simulink model "ECS_Fight_Control_System - Final"  (R2025a)
settings: Solver=ode15s  StartTime=0.0  StopTime=5000  MaxStep=0.1  RelTol=1e-2
libraries: fl_lib x34, nesl_utility x18, SimscapeFluids_lib x8, batt_lib x3, simulink x3, slpidlib x3, simulink_extras x1
(part 1 of 2)
settings Model: SimulationMode=accelerator  Creator=Piyusha  LastModifiedBy=Piyusha

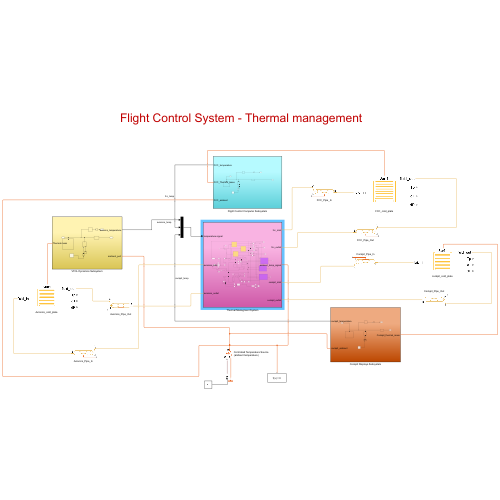
[thumbnail: Simulink's stored preview of the top-level diagram]
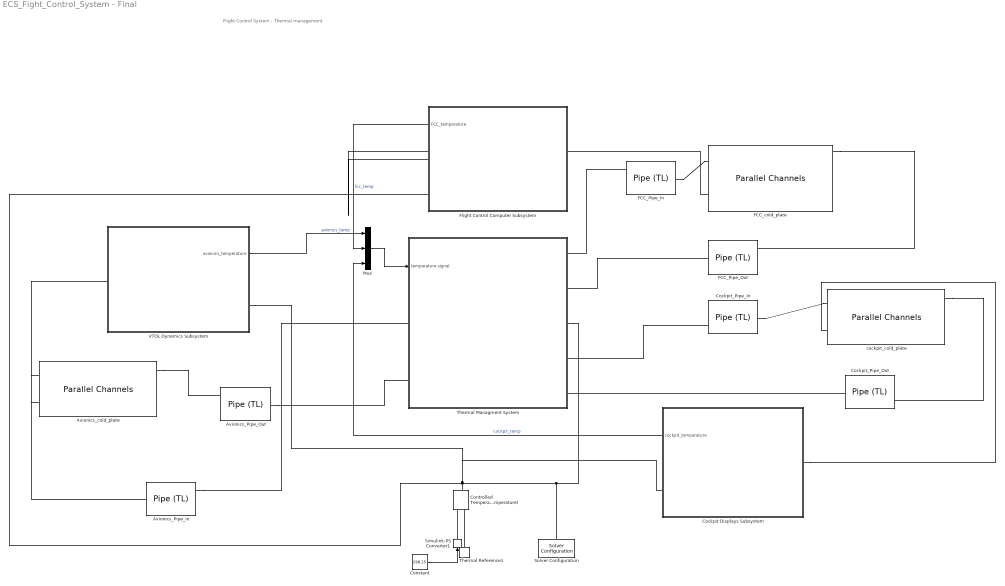
== system ECS_Fight_Control_System - Final ==
  note: Flight Control System - Thermal management
  Avionics_Pipe_In : fl_lib/Thermal Liquid/Elements/Pipe (TL)  length=0.5 m  area=0.006 m^2  Dh=2.827e-5 m  length_add=1 m  roughness=15e-6 m  Re_lam=2000  Re_tur=4000  shape_factor=64  Nu_lam=3.66  dynamic_compressibility=true  inertia=false  p0=0.101325 MPa  T0=298.15 K  mdot0=0 kg/s  p_nominal=0.101325 MPa  T_nominal=293.15 K
  Avionics_Pipe_Out : fl_lib/Thermal Liquid/Elements/Pipe (TL)  length=0.5 m  area=0.006 m^2  Dh=2.827e-5 m  length_add=1 m  roughness=15e-6 m  Re_lam=2000  Re_tur=4000  shape_factor=64  Nu_lam=3.66  dynamic_compressibility=true  inertia=false  p0=0.101325 MPa  T0=298.15 K  mdot0=0 kg/s  p_nominal=0.101325 MPa  T_nominal=293.15 K
  Avionics_cold_plate : batt_lib/Thermal/Parallel Channels  plateConnectivity=simscape.battery.enum.thermal.coolingPlateConnectivity.singleSided  numBattThermalNodes1=1  dimensionThermalNodes1=ones(1, 2)  locationThermalNodes1=ones(1, 2)  numBattThermalNodes2=1  dimensionThermalNodes2=ones(1, 2)  locationThermalNodes2=ones(1, 2)  plateDimX=2  plateDimY=5  plateTh=3e-3 m  plateThCond=200 W/(K*m)  plateDen=2700 kg/m^3  plateCp=900 J/(K*kg)  plateTemp_ini=298.15 K  Re_lam=2000  Re_tur=4000  Nu_lam=3.66  length_add=1e-3 m  shape_factor=64  nChannels=10  selectChannelOrientation=simscape.battery.enum.thermal.coolingChannelsDirection.alongX  channelDia=0.005 m  distributorDia=0.005 m  roughnessPipe=1.5e-05 m
      settings: InternalSimscapePortConfiguration="{\"Bottom\":[],\"Left\":[{\"id\":\"fluid_in\",\"label\":\"fluid_in\",\"type\":\"foundation.thermal_liquid.thermal_liquid\"}],\"Right\":[{\"id\":\"fluid_out\",\"label\":\"fluid_out\",\"type\":\"foundation.thermal_liquid.thermal_liquid\"},{\"id\":\"plotPlateT\",\"label\":\"Tp\",\"type\":\"output\"},{\"id\":\"tempSensor\",\"label\":\"dT\",\"type\":\"output\"},{\"id\":\"presSensor\",\"label\":\"dP\",\"type\":\"output\"}],\"Top\":[{\"id\":\"Side1\",\"label\":\"Surf1\",\"type\":\"foundation.thermal.thermal\"}]}"
  Cockpit Displays Subsystem : Subsystem
  Cockpit_Pipe_In : fl_lib/Thermal Liquid/Elements/Pipe (TL)  length=0.5 m  area=0.006 m^2  Dh=2.827e-5 m  length_add=1 m  roughness=15e-6 m  Re_lam=2000  Re_tur=4000  shape_factor=64  Nu_lam=3.66  dynamic_compressibility=true  inertia=false  p0=0.101325 MPa  T0=298.15 K  mdot0=0 kg/s  p_nominal=0.101325 MPa  T_nominal=293.15 K
  Cockpit_Pipe_Out : fl_lib/Thermal Liquid/Elements/Pipe (TL)  length=0.5 m  area=0.006 m^2  Dh=2.827e-5 m  length_add=1 m  roughness=15e-6 m  Re_lam=2000  Re_tur=4000  shape_factor=64  Nu_lam=3.66  dynamic_compressibility=true  inertia=false  p0=0.101325 MPa  T0=298.15 K  mdot0=0 kg/s  p_nominal=0.101325 MPa  T_nominal=293.15 K
  Constant : Constant  Value=298.15
  Controlled Temperature Source (ambient temperature) : fl_lib/Thermal/Thermal Sources/Controlled Temperature Source
  FCC_Pipe_In : fl_lib/Thermal Liquid/Elements/Pipe (TL)  length=0.5 m  area=0.006 m^2  Dh=2.827e-5 m  length_add=1 m  roughness=15e-6 m  Re_lam=2000  Re_tur=4000  shape_factor=64  Nu_lam=3.66  dynamic_compressibility=true  inertia=false  p0=0.101325 MPa  T0=298.15 K  mdot0=0 kg/s  p_nominal=0.101325 MPa  T_nominal=293.15 K
  FCC_Pipe_Out : fl_lib/Thermal Liquid/Elements/Pipe (TL)  length=0.5 m  area=0.006 m^2  Dh=2.827e-5 m  length_add=1 m  roughness=15e-6 m  Re_lam=2000  Re_tur=4000  shape_factor=64  Nu_lam=3.66  dynamic_compressibility=true  inertia=false  p0=0.101325 MPa  T0=298.15 K  mdot0=0 kg/s  p_nominal=0.101325 MPa  T_nominal=293.15 K
  FCC_cold_plate : batt_lib/Thermal/Parallel Channels  plateConnectivity=simscape.battery.enum.thermal.coolingPlateConnectivity.singleSided  numBattThermalNodes1=1  dimensionThermalNodes1=ones(1, 2)  locationThermalNodes1=ones(1, 2)  numBattThermalNodes2=1  dimensionThermalNodes2=ones(1, 2)  locationThermalNodes2=ones(1, 2)  plateDimX=2  plateDimY=5  plateTh=3e-3 m  plateThCond=200 W/(K*m)  plateDen=2700 kg/m^3  plateCp=900 J/(K*kg)  plateTemp_ini=298.15 K  Re_lam=2000  Re_tur=4000  Nu_lam=3.66  length_add=1e-3 m  shape_factor=64  nChannels=16  selectChannelOrientation=simscape.battery.enum.thermal.coolingChannelsDirection.alongX  channelDia=0.005 m  distributorDia=0.005 m  roughnessPipe=1.5e-05 m
      settings: InternalSimscapePortConfiguration="{\"Bottom\":[],\"Left\":[{\"id\":\"fluid_in\",\"label\":\"fluid_in\",\"type\":\"foundation.thermal_liquid.thermal_liquid\"}],\"Right\":[{\"id\":\"fluid_out\",\"label\":\"fluid_out\",\"type\":\"foundation.thermal_liquid.thermal_liquid\"},{\"id\":\"plotPlateT\",\"label\":\"Tp\",\"type\":\"output\"},{\"id\":\"tempSensor\",\"label\":\"dT\",\"type\":\"output\"},{\"id\":\"presSensor\",\"label\":\"dP\",\"type\":\"output\"}],\"Top\":[{\"id\":\"Side1\",\"label\":\"Surf1\",\"type\":\"foundation.thermal.thermal\"}]}"
  Flight Control Computer Subsystem : Subsystem
  Mux : Mux  Inputs=3
  Simulink-PS Converter1 : nesl_utility/Simulink-PS Converter  PhysicalDomain=network_engine_domain  SubClassName=ps_input  LeftPortType=input  RightPortType=output  PseudoPeriodic=off  Frequencies=[]  NoiseDistribution=none  NoiseParameters=[]  Unit=K  AffineConversion=off  FilteringAndDerivatives=provide  SimscapeFilterOrder=1  InputFilterTimeConstant=0.001  UdotUserProvided=0
  Solver Configuration : nesl_utility/Solver Configuration  PhysicalDomain=network_engine_domain  SubClassName=solver  LeftPortType=input  RightPortType=generic  Tones=[]  Harmonics=[]  SimulateNoise=off  Profile=off  UseLocalSampling=off  EnableSwitchedLinearOptims=on  FrequencyDomain=off  UseCCode=off  RelTol=0.001  AbsTol=0.001  MinStep=1e-09  ToWorkspace=off  RevertToSquareIcSolve=off  NumHomotopyIterations=100  PhasorMode=off  PhasorModeNumHarmonics=1  ConsistencySolver=NEWTON_XTOL_AFTER_FTOL  IndexReductionMethod=DerivativeReplacement  DoDC=off  ResidualTolerance=1e-09  ConsistencyTolSource=GLOBAL  ConsistencyAbsTol=0.001  ConsistencyRelTol=0.001  ConsistencyTolFactor=0.001  UseLocalSolver=off  LocalSolverChoice=NE_BACKWARD_EULER_ADVANCER  ResolveIndetEquations=on  FunctionEvalNumThread=1  LocalSolverSampleTime=0.001  DoFixedCost=off  MaxNonlinIter=3  MaxModeIter=2  ComputeImpulses=off  ImpulseIterations=2  LinearAlgebra=auto  LinearAlgebraNumThread=0  EquationFormulation=NE_TIME_EF  DelaysMemoryBudget=1024  AutomaticFiltering=on  FilteringTimeConstant=0.001  PartitionStorageMethod=AS_NEEDED  PartitionMemoryBudget=1024  PartitionMethod=ROBUST  MultibodyUseLocalSolver=off  MultibodyLocalSolverChoice=ODE1  MultibodyLocalSolverSampleTime=0.001
  Thermal Managment System : Subsystem
  Thermal Reference1 : fl_lib/Thermal/Thermal Elements/Thermal Reference
  VTOL Dynamics Subsystem : Subsystem
  cockpit_cold_plate : batt_lib/Thermal/Parallel Channels  plateConnectivity=simscape.battery.enum.thermal.coolingPlateConnectivity.singleSided  numBattThermalNodes1=1  dimensionThermalNodes1=ones(1, 2)  locationThermalNodes1=ones(1, 2)  numBattThermalNodes2=1  dimensionThermalNodes2=ones(1, 2)  locationThermalNodes2=ones(1, 2)  plateDimX=2  plateDimY=5  plateTh=3e-3 m  plateThCond=200 W/(K*m)  plateDen=2700 kg/m^3  plateCp=900 J/(K*kg)  plateTemp_ini=298.15 K  Re_lam=2000  Re_tur=4000  Nu_lam=3.66  length_add=1e-3 m  shape_factor=64  nChannels=24  selectChannelOrientation=simscape.battery.enum.thermal.coolingChannelsDirection.alongX  channelDia=0.005 m  distributorDia=0.005 m  roughnessPipe=1.5e-05 m
      settings: InternalSimscapePortConfiguration="{\"Bottom\":[],\"Left\":[{\"id\":\"fluid_in\",\"label\":\"fluid_in\",\"type\":\"foundation.thermal_liquid.thermal_liquid\"}],\"Right\":[{\"id\":\"fluid_out\",\"label\":\"fluid_out\",\"type\":\"foundation.thermal_liquid.thermal_liquid\"},{\"id\":\"plotPlateT\",\"label\":\"Tp\",\"type\":\"output\"},{\"id\":\"tempSensor\",\"label\":\"dT\",\"type\":\"output\"},{\"id\":\"presSensor\",\"label\":\"dP\",\"type\":\"output\"}],\"Top\":[{\"id\":\"Side1\",\"label\":\"Surf1\",\"type\":\"foundation.thermal.thermal\"}]}"
  wires:
  Flight Control Computer Subsystem/1(FCC_temperature) -> Mux/2  "fcc_temp"
  Cockpit Displays Subsystem/1(cockpit_temperature) -> Mux/3  "cockpit_temp"
  VTOL Dynamics Subsystem/1(avionics_temperature) -> Mux/1  "avionics_temp"
  Mux/1 -> Thermal Managment System/1(temperature signal)
  Constant/1 -> Simulink-PS Converter1/1
  connections:
  Thermal Reference1/LConn1 -- Controlled Temperature Source (ambient temperature)/RConn2
  Simulink-PS Converter1/RConn1 -- Controlled Temperature Source (ambient temperature)/RConn1
  Thermal Managment System/RConn3 -- VTOL Dynamics Subsystem/RConn1 -- Cockpit Displays Subsystem/RConn1 -- Controlled Temperature Source (ambient temperature)/LConn1 -- Flight Control Computer Subsystem/RConn2 -- Solver Configuration/RConn1
  Avionics_cold_plate/LConn2 -- VTOL Dynamics Subsystem/LConn1
  Avionics_Pipe_In/RConn1 -- Avionics_cold_plate/LConn1
  Avionics_cold_plate/RConn1 -- Avionics_Pipe_Out/LConn1
  Avionics_Pipe_In/LConn1 -- Thermal Managment System/LConn1
  Avionics_Pipe_Out/RConn1 -- Thermal Managment System/LConn2
  FCC_Pipe_In/RConn1 -- FCC_cold_plate/LConn1
  FCC_cold_plate/RConn1 -- FCC_Pipe_Out/LConn1
  FCC_Pipe_In/LConn1 -- Thermal Managment System/RConn1
  FCC_Pipe_Out/RConn1 -- Thermal Managment System/RConn2
  Cockpit_Pipe_In/RConn1 -- cockpit_cold_plate/LConn1
  cockpit_cold_plate/RConn1 -- Cockpit_Pipe_Out/LConn1
  Cockpit_Pipe_In/LConn1 -- Thermal Managment System/RConn4
  Cockpit_Pipe_Out/RConn1 -- Thermal Managment System/RConn5
  Cockpit Displays Subsystem/LConn1 -- cockpit_cold_plate/LConn2
  FCC_cold_plate/LConn2 -- Flight Control Computer Subsystem/RConn1

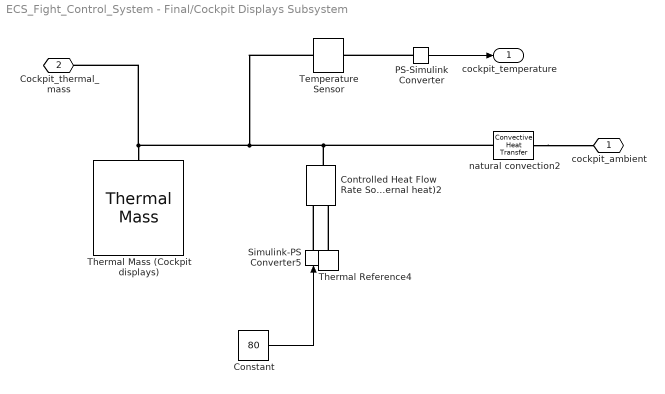
== system ECS_Fight_Control_System - Final/Cockpit Displays Subsystem ==
  Constant : Constant  Value=80
  Controlled Heat Flow Rate Source (Internal heat)2 : fl_lib/Thermal/Thermal Sources/Controlled Heat Flow Rate Source
  PS-Simulink Converter : nesl_utility/PS-Simulink Converter  PhysicalDomain=network_engine_domain  SubClassName=ps_output  LeftPortType=input  RightPortType=output  PseudoPeriodic=off  Frequencies=[]  VectorFormat=inherit  Unit=inherit  AffineConversion=off
  Simulink-PS Converter5 : nesl_utility/Simulink-PS Converter  PhysicalDomain=network_engine_domain  SubClassName=ps_input  LeftPortType=input  RightPortType=output  PseudoPeriodic=off  Frequencies=[]  NoiseDistribution=none  NoiseParameters=[]  Unit=W  AffineConversion=off  FilteringAndDerivatives=provide  SimscapeFilterOrder=1  InputFilterTimeConstant=0.001  UdotUserProvided=0
  Temperature Sensor : fl_lib/Thermal/Thermal Sensors/Temperature Sensor  temperature_measure=foundation.enum.MeasurementReference.absolute
      settings: InternalSimscapePortConfiguration="{\"Bottom\":[],\"Left\":[{\"id\":\"A\",\"label\":\"A\",\"type\":\"foundation.thermal.thermal\"}],\"Right\":[{\"id\":\"T\",\"label\":\"T\",\"type\":\"output\"}],\"Top\":[]}"
  Thermal Mass (Cockpit displays) : fl_lib/Thermal/Thermal Elements/Thermal Mass  mass_type=foundation.enum.constant_variable.constant  mass=13 kg  sp_heat=900 J/(K*kg)  mass_min=1e-6 kg  num_ports=foundation.enum.numPorts2.one  m_specify=off  m_priority=High  m=1 kg  m_nominal_specify=off  m_nominal_value=1  m_nominal_unit=kg  T_specify=on  T_priority=None  T=312 K  T_nominal_specify=off  T_nominal_value=350  T_nominal_unit=K  Q_specify=off  Q_priority=None  Q=0 W  Q_nominal_specify=off  Q_nominal_value=1  Q_nominal_unit=W
  Thermal Reference4 : fl_lib/Thermal/Thermal Elements/Thermal Reference
  natural convection2 : fl_lib/Thermal/Thermal Elements/Convective Heat Transfer  thermal_type=foundation.enum.constant_variable.constant  area=0.3 m^2  heat_tr_coeff=10 W/(K*m^2)  min_heat_tr_coeff=1e-3 W/(K*m^2)  T_specify=off  T_priority=None  T=0 K  T_nominal_specify=off  T_nominal_value=1  T_nominal_unit=K  Q_specify=off  Q_priority=None  Q=0 W  Q_nominal_specify=off  Q_nominal_value=1  Q_nominal_unit=W
  cockpit_ambient : PMIOPort  Side=Right
  Cockpit_thermal_mass : PMIOPort  Port=2  Side=Left
  cockpit_temperature : Outport
  wires:
  PS-Simulink Converter/1 -> cockpit_temperature/1
  Constant/1 -> Simulink-PS Converter5/1
  connections:
  natural convection2/RConn1 -- cockpit_ambient/RConn1
  Controlled Heat Flow Rate Source (Internal heat)2/LConn1 -- natural convection2/LConn1 -- Temperature Sensor/LConn1 -- Cockpit_thermal_mass/RConn1 -- Thermal Mass (Cockpit displays)/LConn1
  Simulink-PS Converter5/RConn1 -- Controlled Heat Flow Rate Source (Internal heat)2/RConn1
  Thermal Reference4/LConn1 -- Controlled Heat Flow Rate Source (Internal heat)2/RConn2
  PS-Simulink Converter/LConn1 -- Temperature Sensor/RConn1

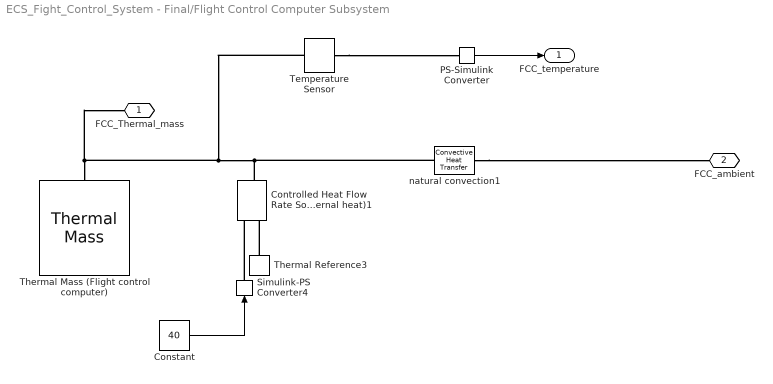
== system ECS_Fight_Control_System - Final/Flight Control Computer Subsystem ==
  Constant : Constant  Value=40
  Controlled Heat Flow Rate Source (Internal heat)1 : fl_lib/Thermal/Thermal Sources/Controlled Heat Flow Rate Source
  PS-Simulink Converter : nesl_utility/PS-Simulink Converter  PhysicalDomain=network_engine_domain  SubClassName=ps_output  LeftPortType=input  RightPortType=output  PseudoPeriodic=off  Frequencies=[]  VectorFormat=inherit  Unit=inherit  AffineConversion=off
  Simulink-PS Converter4 : nesl_utility/Simulink-PS Converter  PhysicalDomain=network_engine_domain  SubClassName=ps_input  LeftPortType=input  RightPortType=output  PseudoPeriodic=off  Frequencies=[]  NoiseDistribution=none  NoiseParameters=[]  Unit=W  AffineConversion=off  FilteringAndDerivatives=provide  SimscapeFilterOrder=1  InputFilterTimeConstant=0.001  UdotUserProvided=0
  Temperature Sensor : fl_lib/Thermal/Thermal Sensors/Temperature Sensor  temperature_measure=foundation.enum.MeasurementReference.absolute
      settings: InternalSimscapePortConfiguration="{\"Bottom\":[],\"Left\":[{\"id\":\"A\",\"label\":\"A\",\"type\":\"foundation.thermal.thermal\"}],\"Right\":[{\"id\":\"T\",\"label\":\"T\",\"type\":\"output\"}],\"Top\":[]}"
  Thermal Mass (Flight control computer) : fl_lib/Thermal/Thermal Elements/Thermal Mass  mass_type=foundation.enum.constant_variable.constant  mass=4.5 kg  sp_heat=900 J/(K*kg)  mass_min=1e-6 kg  num_ports=foundation.enum.numPorts2.one  m_specify=off  m_priority=High  m=1 kg  m_nominal_specify=off  m_nominal_value=1  m_nominal_unit=kg  T_specify=on  T_priority=None  T=310 K  T_nominal_specify=off  T_nominal_value=350  T_nominal_unit=K  Q_specify=off  Q_priority=None  Q=0 W  Q_nominal_specify=off  Q_nominal_value=1  Q_nominal_unit=W
  Thermal Reference3 : fl_lib/Thermal/Thermal Elements/Thermal Reference
  natural convection1 : fl_lib/Thermal/Thermal Elements/Convective Heat Transfer  thermal_type=foundation.enum.constant_variable.constant  area=0.22 m^2  heat_tr_coeff=10 W/(K*m^2)  min_heat_tr_coeff=1e-3 W/(K*m^2)  T_specify=off  T_priority=None  T=0 K  T_nominal_specify=off  T_nominal_value=1  T_nominal_unit=K  Q_specify=off  Q_priority=None  Q=0 W  Q_nominal_specify=off  Q_nominal_value=1  Q_nominal_unit=W
  FCC_Thermal_mass : PMIOPort  Side=Right
  FCC_ambient : PMIOPort  Port=2  Side=Right
  FCC_temperature : Outport
  wires:
  PS-Simulink Converter/1 -> FCC_temperature/1
  Constant/1 -> Simulink-PS Converter4/1
  connections:
  Thermal Reference3/LConn1 -- Controlled Heat Flow Rate Source (Internal heat)1/RConn2
  Simulink-PS Converter4/RConn1 -- Controlled Heat Flow Rate Source (Internal heat)1/RConn1
  natural convection1/LConn1 -- Temperature Sensor/LConn1 -- FCC_Thermal_mass/RConn1 -- Thermal Mass (Flight control computer)/LConn1 -- Controlled Heat Flow Rate Source (Internal heat)1/LConn1
  natural convection1/RConn1 -- FCC_ambient/RConn1
  Temperature Sensor/RConn1 -- PS-Simulink Converter/LConn1

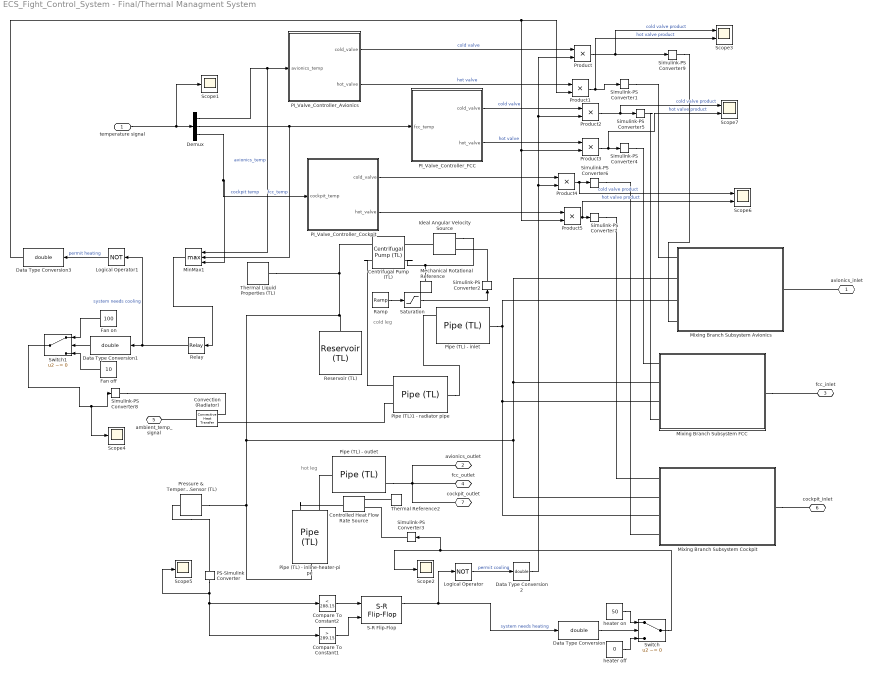
== system ECS_Fight_Control_System - Final/Thermal Managment System ==
  note: cold leg
  note: hot leg
  temperature signal : Inport
  Centrifugal Pump (TL) : SimscapeFluids_lib/Thermal Liquid/Pumps & Motors/Centrifugal Pump (TL)  pump_parameterization=fluids.thermal_liquid.pumps_motors.enum.CentrifugalPumpParameterization.Nominal  capacity_ref_nominal=5 lpm  head_ref_nominal=4 m  power_ref_nominal=0.02 kW  head_ref_max=8 m  capacity_ref_max=8 lpm  omega_ref_analytic=3000 rpm  flow_rate_1D_TLU=[16.67, 30, 40, 53.33, 66.67, 83.33] lpm  head_1D_TLU=[50, 47.5, 45, 40, 35, 25] m  power_1D_TLU=[.6, .75, .85, .93, .98, .99] kW  omega_ref_1D=3500 rpm  rho_ref_1D=998.21 kg/m^3  omega_threshold_factor=1e-2  flow_rate_2D_TLU=[16.67, 23.33, 30, 40, 53.33, 60] lpm  omega_2D_TLU=[2450, 2800, 3150, 3500] rpm  head_2D_TLU=[25, 32.7, 42.5, 50; 24, 31.7, 41, 49; 22.7, 30.5, 39, 47.5; 20, 28, 36, 45; 15.7, 24, 32, 40; 12.5, 21, 29.5, 37.5] m  power_2D_TLU=[.28, .38, .5, .6; .31, .41, .55, .68; .33, .44, .6, .75; .36, .48, .65, .83; .38, .53, .72, .93; .39, .55, .75, .97] kW  rho_ref_2D=998.21 kg/m^3  diameter_ratio=1  mech_orientation=fluids.thermal_liquid.pumps_motors.enum.CentrifugalPumpMechOrientation.Positive  area=7.854e-5 m^2  operation_check=simscape.enum.assert.action.none
      settings: InternalSimscapePortConfiguration="{\"Bottom\":[],\"Left\":[{\"id\":\"A\",\"label\":\"A\",\"type\":\"foundation.thermal_liquid.thermal_liquid\"},{\"id\":\"B\",\"label\":\"B\",\"type\":\"foundation.thermal_liquid.thermal_liquid\"}],\"Right\":[{\"id\":\"R\",\"label\":\"R\",\"type\":\"foundation.mechanical.rotational.rotational\"},{\"id\":\"C\",\"label\":\"C\",\"type\":\"foundation.mechanical.rotational.rotational\"}],\"Top\":[]}"
  Compare To Constant1 : simulink/Logic and Bit Operations/Compare To Constant  relop=>  const=289.15  OutDataTypeStr=boolean
  Compare To Constant2 : simulink/Logic and Bit Operations/Compare To Constant  relop=<  const=288.15  OutDataTypeStr=boolean
  Controlled Heat Flow Rate Source : fl_lib/Thermal/Thermal Sources/Controlled Heat Flow Rate Source
  Convection (Radiator) : fl_lib/Thermal/Thermal Elements/Convective Heat Transfer  thermal_type=foundation.enum.constant_variable.variable  area=0.5 m^2  heat_tr_coeff=100 W/(K*m^2)  min_heat_tr_coeff=1e-3 W/(K*m^2)  T_specify=off  T_priority=None  T=0 K  T_nominal_specify=off  T_nominal_value=1  T_nominal_unit=K  Q_specify=off  Q_priority=None  Q=0 W  Q_nominal_specify=off  Q_nominal_value=1  Q_nominal_unit=W
      settings: InternalSimscapePortConfiguration="{\"Bottom\":[],\"Left\":[{\"id\":\"A\",\"label\":\"A\",\"type\":\"foundation.thermal.thermal\"},{\"id\":\"var_heat_tr_coeff\",\"label\":\"K\",\"type\":\"input\"}],\"Right\":[{\"id\":\"B\",\"label\":\"B\",\"type\":\"foundation.thermal.thermal\"}],\"Top\":[]}"
  Data Type Conversion{,1..3} (4 alike) : DataTypeConversion  OutDataTypeStr=double  SaturateOnIntegerOverflow=off  RndMeth=Floor
  Demux : Demux  Outputs=3
  Fan off : Constant  Value=10
  Fan on : Constant  Value=100
  Ideal Angular Velocity Source : fl_lib/Mechanical/Mechanical Sources/Ideal Angular Velocity Source
  Logical Operator : Logic  Operator=NOT  AllPortsSameDT=off  OutDataTypeStr=boolean
  Logical Operator1 : Logic  Operator=NOT  AllPortsSameDT=off  OutDataTypeStr=boolean
  Mechanical Rotational Reference : fl_lib/Mechanical/Rotational Elements/Mechanical Rotational Reference
  MinMax1 : MinMax  Function=max  Inputs=3
  Mixing Branch Subsystem Avionics : Subsystem
  Mixing Branch Subsystem Cockpit : Subsystem
  Mixing Branch Subsystem FCC : Subsystem
  PI_Valve_Controller_Avionics : Subsystem
  PI_Valve_Controller_Cockpit : Subsystem
  PI_Valve_Controller_FCC : Subsystem
  PS-Simulink Converter : nesl_utility/PS-Simulink Converter  PhysicalDomain=network_engine_domain  SubClassName=ps_output  LeftPortType=input  RightPortType=output  PseudoPeriodic=off  Frequencies=[]  VectorFormat=inherit  Unit=inherit  AffineConversion=off
  Pipe (TL) - inlet : fl_lib/Thermal Liquid/Elements/Pipe (TL)  length=1.5 m  area=7.854e-5 m^2  Dh=0.01 m  length_add=1 m  roughness=15e-6 m  Re_lam=2000  Re_tur=4000  shape_factor=64  Nu_lam=3.66  dynamic_compressibility=true  inertia=false  p0=0.101325 MPa  T0=298.15 K  mdot0=0 kg/s  p_nominal=0.101325 MPa  T_nominal=293.15 K
  Pipe (TL) - inline-heater-pipe : fl_lib/Thermal Liquid/Elements/Pipe (TL)  length=0.1 m  area=7.854e-5 m^2  Dh=0.01 m  length_add=1 m  roughness=15e-6 m  Re_lam=2000  Re_tur=4000  shape_factor=64  Nu_lam=3.66  dynamic_compressibility=true  inertia=false  p0=0.101325 MPa  T0=298.15 K  mdot0=0 kg/s  p_nominal=0.101325 MPa  T_nominal=293.15 K
  Pipe (TL) - outlet : fl_lib/Thermal Liquid/Elements/Pipe (TL)  length=1.5 m  area=7.854e-5 m^2  Dh=0.01 m  length_add=1 m  roughness=15e-6 m  Re_lam=2000  Re_tur=4000  shape_factor=64  Nu_lam=3.66  dynamic_compressibility=true  inertia=false  p0=0.101325 MPa  T0=298.15 K  mdot0=0 kg/s  p_nominal=0.101325 MPa  T_nominal=293.15 K
  Pipe (TL)1 - radiator pipe : fl_lib/Thermal Liquid/Elements/Pipe (TL)  length=0.75 m  area=7.854e-5 m^2  Dh=0.01 m  length_add=1 m  roughness=15e-6 m  Re_lam=2000  Re_tur=4000  shape_factor=64  Nu_lam=3.66  dynamic_compressibility=true  inertia=false  p0=0.101325 MPa  T0=298.15 K  mdot0=0 kg/s  p_nominal=0.101325 MPa  T_nominal=293.15 K
  Pressure & Temperature Sensor (TL) : fl_lib/Thermal Liquid/Sensors/Pressure & Temperature Sensor (TL)  reference=foundation.enum.MeasurementReference.absolute  pressure=false  pressure_spec=foundation.enum.PressureMeasementSpec.Absolute  temperature=true
      settings: InternalSimscapePortConfiguration="{\"Bottom\":[{\"id\":\"T\",\"label\":\"T\",\"type\":\"output\"}],\"Left\":[{\"id\":\"A\",\"label\":\"A\",\"type\":\"foundation.thermal_liquid.thermal_liquid\"}],\"Right\":[],\"Top\":[]}"
  Product{,1..5} (6 alike) : Product
  Ramp : simulink/Sources/Ramp  slope=1000  start=1  InitialOutput=0
  Relay : Relay  OnSwitchValue=308.15  OffSwitchValue=307.15
  "Reservoir (TL) " : fl_lib/Thermal Liquid/Elements/Reservoir (TL)  pressure_spec=foundation.enum.pressure_spec.atmospheric  reservoir_pressure=0.101325 MPa  reservoir_temperature=298.15 K  area=7.854e-5 m^2
  S-R Flip-Flop : simulink_extras/Flip Flops/S-R Flip-Flop  initial_condition=0
  Saturation : Saturate  UpperLimit=3000  LowerLimit=0
  Scope{1..2,4..5} (4 alike) : Scope
      Scope1 settings: ActiveDisplayYMinimum=294.34876570244938  ActiveDisplayYMaximum=309.81465883467445
      Scope2 settings: ActiveDisplayYMinimum=-18.574706388101248  ActiveDisplayYMaximum=67.656527037864834  DataLoggingVariableName=ScopeData2
      Scope4 settings: ActiveDisplayYMinimum=-17.443836096573261  ActiveDisplayYMaximum=62.456397666600694  DataLoggingVariableName=ScopeData4
      Scope5 settings: ActiveDisplayYMinimum=292.31370524419793  ActiveDisplayYMaximum=296.28099923951214  DataLoggingVariableName=ScopeData5
  Scope3 : Scope  NumInputPorts=2
      settings: ActiveDisplayYMinimum=-0.24217564391764534  ActiveDisplayYMaximum=0.68337651791294018  DataLoggingVariableName=ScopeData3
  Scope6 : Scope  NumInputPorts=2
      settings: ActiveDisplayYMinimum=-0.26550876950504732  ActiveDisplayYMaximum=1.3314895720023909  DataLoggingVariableName=ScopeData6
  Scope7 : Scope  NumInputPorts=2
      settings: ActiveDisplayYMinimum=-0.25040000463615819  ActiveDisplayYMaximum=1.2618169694914934
  Simulink-PS Converter{1,4..7,9} (6 alike) : nesl_utility/Simulink-PS Converter  PhysicalDomain=network_engine_domain  SubClassName=ps_input  LeftPortType=input  RightPortType=output  PseudoPeriodic=off  Frequencies=[]  NoiseDistribution=none  NoiseParameters=[]  Unit=1  AffineConversion=off  FilteringAndDerivatives=provide  SimscapeFilterOrder=1  InputFilterTimeConstant=0.001  UdotUserProvided=0
  Simulink-PS Converter2 : nesl_utility/Simulink-PS Converter  PhysicalDomain=network_engine_domain  SubClassName=ps_input  LeftPortType=input  RightPortType=output  PseudoPeriodic=off  Frequencies=[]  NoiseDistribution=none  NoiseParameters=[]  Unit=rpm  AffineConversion=off  FilteringAndDerivatives=provide  SimscapeFilterOrder=1  InputFilterTimeConstant=0.001  UdotUserProvided=0
  Simulink-PS Converter3 : nesl_utility/Simulink-PS Converter  PhysicalDomain=network_engine_domain  SubClassName=ps_input  LeftPortType=input  RightPortType=output  PseudoPeriodic=off  Frequencies=[]  NoiseDistribution=none  NoiseParameters=[]  Unit=W  AffineConversion=off  FilteringAndDerivatives=provide  SimscapeFilterOrder=1  InputFilterTimeConstant=0.001  UdotUserProvided=0
  Simulink-PS Converter8 : nesl_utility/Simulink-PS Converter  PhysicalDomain=network_engine_domain  SubClassName=ps_input  LeftPortType=input  RightPortType=output  PseudoPeriodic=off  Frequencies=[]  NoiseDistribution=none  NoiseParameters=[]  Unit=W/(m^2*K)  AffineConversion=off  FilteringAndDerivatives=provide  SimscapeFilterOrder=1  InputFilterTimeConstant=0.001  UdotUserProvided=0
  Switch : Switch  Criteria=u2 ~= 0  SaturateOnIntegerOverflow=off  InputSameDT=off
  Switch1 : Switch  Criteria=u2 ~= 0  SaturateOnIntegerOverflow=off  InputSameDT=off
  "Thermal Liquid Properties (TL) " : SimscapeFluids_lib/Thermal Liquid/Utilities/Thermal Liquid Properties (TL)  fluid_list=fluids.thermal_liquid.utilities.enum.thermal_liquid_fluid_list.ethylene_glycol  concentration_param_EG=fluids.thermal_liquid.utilities.enum.thermal_liquid_concentration.volume_fraction  concentration_param_PG=fluids.thermal_liquid.utilities.enum.thermal_liquid_concentration.volume_fraction  c_mass_SW=3.5e-3  c_mass_EG=0.1  c_mass_PG=0.1  c_mass_GL=0.1  c_vol_EG=0.6  c_vol_PG=0.1  beta_const_EG=2.1791 GPa  beta_const_PG=2.1791 GPa  beta_const_GL=2.1791 GPa  p_min_EG=0.01 MPa  p_min_PG=0.01 MPa  p_min_GL=0.01 MPa  p_max_EG=50 MPa  p_max_PG=50 MPa  p_max_GL=50 MPa  p_atm=0.101325 MPa  properties_range_check=simscape.enum.assert.action.error
  Thermal Reference2 : fl_lib/Thermal/Thermal Elements/Thermal Reference
  heater off : Constant  Value=0
  heater on : Constant  Value=50
  avionics_inlet : PMIOPort  Side=Left
  avionics_outlet : PMIOPort  Port=2  Side=Left
  fcc_inlet : PMIOPort  Port=3  Side=Right
  fcc_outlet : PMIOPort  Port=4  Side=Right
  ambient_temp_signal : PMIOPort  Port=5  Side=Right
  cockpit_inlet : PMIOPort  Port=6  Side=Right
  cockpit_outlet : PMIOPort  Port=7  Side=Right
  wires:
  temperature signal/1 -> Scope1/1, Demux/1
  Demux/1 -> MinMax1/1, PI_Valve_Controller_Avionics/1(avionics_temp)  "avionics_temp"
  Demux/2 -> MinMax1/2, PI_Valve_Controller_FCC/1(fcc_temp)  "fcc_temp"
  Saturation/1 -> Simulink-PS Converter2/1
  Data Type Conversion/1 -> Switch/2
  heater on/1 -> Switch/1
  heater off/1 -> Switch/3
  Data Type Conversion1/1 -> Switch1/2
  Fan on/1 -> Switch1/1
  Fan off/1 -> Switch1/3
  Compare To Constant2/1 -> S-R Flip-Flop/1
  Compare To Constant1/1 -> S-R Flip-Flop/2
  Switch1/1 -> Scope4/1, Simulink-PS Converter8/1
  Switch/1 -> Simulink-PS Converter3/1, Scope2/1
  PI_Valve_Controller_Avionics/1(cold_valve) -> Product/1  "cold valve"
  S-R Flip-Flop/1 -> Data Type Conversion/1, Logical Operator/1  "system needs heating"
  Relay/1 -> Logical Operator1/1, Data Type Conversion1/1  "system needs cooling"
  MinMax1/1 -> Relay/1
  Logical Operator/1 -> Data Type Conversion2/1  "permit cooling"
  Logical Operator1/1 -> Data Type Conversion3/1  "permit heating"
  Product/1 -> Scope3/1, Simulink-PS Converter9/1  "cold valve product"
  Data Type Conversion3/1 -> Product1/2, Product3/2, Product5/2
  PI_Valve_Controller_Avionics/2(hot_valve) -> Product1/1  "hot valve"
  Product1/1 -> Scope3/2, Simulink-PS Converter1/1  "hot valve product"
  Data Type Conversion2/1 -> Product2/2, Product/2, Product4/2
  PI_Valve_Controller_FCC/1(cold_valve) -> Product2/1  "cold valve"
  Product2/1 -> Scope7/1, Simulink-PS Converter5/1  "cold valve product"
  PI_Valve_Controller_FCC/2(hot_valve) -> Product3/1  "hot valve"
  Product3/1 -> Scope7/2, Simulink-PS Converter4/1  "hot valve product"
  Demux/3 -> PI_Valve_Controller_Cockpit/1(cockpit_temp), MinMax1/3  "cockpit temp"
  PI_Valve_Controller_Cockpit/1(cold_valve) -> Product4/1
  PI_Valve_Controller_Cockpit/2(hot_valve) -> Product5/1
  Product4/1 -> Scope6/1, Simulink-PS Converter6/1  "cold valve product"
  Product5/1 -> Scope6/2, Simulink-PS Converter7/1  "hot valve product"
  PS-Simulink Converter/1 -> Scope5/1, Compare To Constant2/1, Compare To Constant1/1
  Ramp/1 -> Saturation/1
  connections:
  "Thermal Liquid Properties (TL) "/RConn1 -- Pressure & Temperature Sensor (TL)/LConn1 -- Pipe (TL) - inline-heater-pipe/RConn1 -- Mixing Branch Subsystem Avionics/LConn2 -- Mixing Branch Subsystem FCC/LConn2 -- Mixing Branch Subsystem Cockpit/LConn2 -- "Reservoir (TL) "/LConn1 -- Centrifugal Pump (TL)/LConn1
  Simulink-PS Converter2/RConn1 -- Ideal Angular Velocity Source/RConn1
  Thermal Reference2/LConn1 -- Controlled Heat Flow Rate Source/RConn2
  Ideal Angular Velocity Source/LConn1 -- Centrifugal Pump (TL)/RConn1
  Centrifugal Pump (TL)/RConn2 -- Ideal Angular Velocity Source/RConn2 -- Mechanical Rotational Reference/LConn1
  Pipe (TL)1 - radiator pipe/LConn2 -- Convection (Radiator)/LConn1
  Convection (Radiator)/RConn1 -- ambient_temp_signal/RConn1
  Simulink-PS Converter3/RConn1 -- Controlled Heat Flow Rate Source/RConn1
  Centrifugal Pump (TL)/LConn2 -- Pipe (TL)1 - radiator pipe/LConn1
  Pipe (TL) - outlet/RConn1 -- Pipe (TL) - inline-heater-pipe/LConn1
  Pipe (TL)1 - radiator pipe/RConn1 -- Pipe (TL) - inlet/LConn1
  Pipe (TL) - outlet/LConn1 -- cockpit_outlet/RConn1 -- avionics_outlet/RConn1 -- fcc_outlet/RConn1
  avionics_inlet/RConn1 -- Mixing Branch Subsystem Avionics/RConn1
  Pipe (TL) - inlet/RConn1 -- Mixing Branch Subsystem FCC/LConn3 -- Mixing Branch Subsystem Cockpit/LConn3 -- Mixing Branch Subsystem Avionics/LConn3
  Pipe (TL) - inline-heater-pipe/LConn2 -- Controlled Heat Flow Rate Source/LConn1
  Mixing Branch Subsystem FCC/RConn1 -- fcc_inlet/RConn1
  Mixing Branch Subsystem Cockpit/RConn1 -- cockpit_inlet/RConn1
  Simulink-PS Converter1/RConn1 -- Mixing Branch Subsystem Avionics/LConn1
  Simulink-PS Converter5/RConn1 -- Mixing Branch Subsystem FCC/LConn4
  Simulink-PS Converter4/RConn1 -- Mixing Branch Subsystem FCC/LConn1
  Simulink-PS Converter6/RConn1 -- Mixing Branch Subsystem Cockpit/LConn4
  Simulink-PS Converter7/RConn1 -- Mixing Branch Subsystem Cockpit/LConn1
  Simulink-PS Converter8/RConn1 -- Convection (Radiator)/LConn2
  Simulink-PS Converter9/RConn1 -- Mixing Branch Subsystem Avionics/LConn4
  Pressure & Temperature Sensor (TL)/RConn1 -- PS-Simulink Converter/LConn1

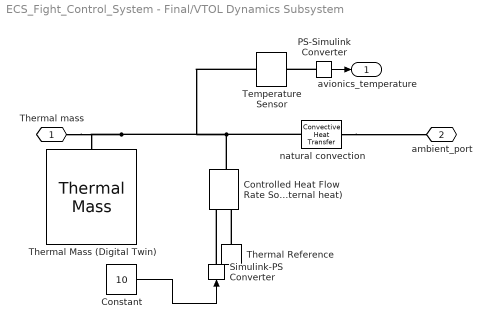
== system ECS_Fight_Control_System - Final/VTOL Dynamics Subsystem ==
  Constant : Constant  Value=10
  Controlled Heat Flow Rate Source (Internal heat) : fl_lib/Thermal/Thermal Sources/Controlled Heat Flow Rate Source
  PS-Simulink Converter : nesl_utility/PS-Simulink Converter  PhysicalDomain=network_engine_domain  SubClassName=ps_output  LeftPortType=input  RightPortType=output  PseudoPeriodic=off  Frequencies=[]  VectorFormat=inherit  Unit=inherit  AffineConversion=off
  Simulink-PS Converter : nesl_utility/Simulink-PS Converter  PhysicalDomain=network_engine_domain  SubClassName=ps_input  LeftPortType=input  RightPortType=output  PseudoPeriodic=off  Frequencies=[]  NoiseDistribution=none  NoiseParameters=[]  Unit=W  AffineConversion=off  FilteringAndDerivatives=provide  SimscapeFilterOrder=1  InputFilterTimeConstant=0.001  UdotUserProvided=0
  Temperature Sensor : fl_lib/Thermal/Thermal Sensors/Temperature Sensor  temperature_measure=foundation.enum.MeasurementReference.absolute
      settings: InternalSimscapePortConfiguration="{\"Bottom\":[],\"Left\":[{\"id\":\"A\",\"label\":\"A\",\"type\":\"foundation.thermal.thermal\"}],\"Right\":[{\"id\":\"T\",\"label\":\"T\",\"type\":\"output\"}],\"Top\":[]}"
  Thermal Mass (Digital Twin) : fl_lib/Thermal/Thermal Elements/Thermal Mass  mass_type=foundation.enum.constant_variable.constant  mass=1.2 kg  sp_heat=900 J/(K*kg)  mass_min=1e-6 kg  num_ports=foundation.enum.numPorts2.one  m_specify=off  m_priority=High  m=1 kg  m_nominal_specify=off  m_nominal_value=1  m_nominal_unit=kg  T_specify=on  T_priority=High  T=283 K  T_nominal_specify=off  T_nominal_value=350  T_nominal_unit=K  Q_specify=off  Q_priority=None  Q=0 W  Q_nominal_specify=off  Q_nominal_value=1  Q_nominal_unit=W
  Thermal Reference : fl_lib/Thermal/Thermal Elements/Thermal Reference
  natural convection : fl_lib/Thermal/Thermal Elements/Convective Heat Transfer  thermal_type=foundation.enum.constant_variable.constant  area=0.04 m^2  heat_tr_coeff=10 W/(K*m^2)  min_heat_tr_coeff=1e-3 W/(K*m^2)  T_specify=off  T_priority=None  T=0 K  T_nominal_specify=off  T_nominal_value=1  T_nominal_unit=K  Q_specify=off  Q_priority=None  Q=0 W  Q_nominal_specify=off  Q_nominal_value=1  Q_nominal_unit=W
  Thermal mass : PMIOPort  Side=Left
  ambient_port : PMIOPort  Port=2  Side=Right
  avionics_temperature : Outport
  wires:
  PS-Simulink Converter/1 -> avionics_temperature/1
  Constant/1 -> Simulink-PS Converter/1
  connections:
  Thermal Reference/LConn1 -- Controlled Heat Flow Rate Source (Internal heat)/RConn2
  PS-Simulink Converter/LConn1 -- Temperature Sensor/RConn1
  natural convection/RConn1 -- ambient_port/RConn1
  Simulink-PS Converter/RConn1 -- Controlled Heat Flow Rate Source (Internal heat)/RConn1
  Controlled Heat Flow Rate Source (Internal heat)/LConn1 -- natural convection/LConn1 -- Thermal Mass (Digital Twin)/LConn1 -- Thermal mass/RConn1 -- Temperature Sensor/LConn1

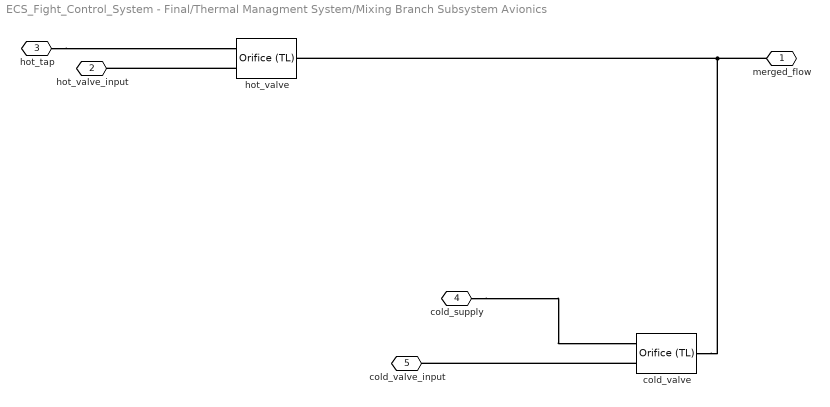
== system ECS_Fight_Control_System - Final/Thermal Managment System/Mixing Branch Subsystem Avionics ==
  cold_valve : SimscapeFluids_lib/Thermal Liquid/Valves & Orifices/Orifice (TL)  orifice_type=foundation.enum.constant_variable.variable  constant_orifice_spec=fluids.thermal_liquid.valves.enum.ConstantOrificeSpec.Area  variable_orifice_spec=fluids.thermal_liquid.valves.enum.orifice_spec.linear  orifice_area_constant=1e-3 m^2  p_diff_TLU_constant=[-4, -3, -2, -1, -.5, 0, .5, 1, 2, 3, 4] MPa  vol_flow_TLU_constant=[-2.44, -2.12, -1.68, -1.22, -.84, 0, .85, 1.21, 1.7, 2.09, 2.41] .* 1e-3 m^3/s  mdot_TLU_constant=[-2.44, -2.12, -1.68, -1.22, -.84, 0, .85, 1.21, 1.7, 2.09, 2.41] kg/s  S_min=0 m  del_S=5e-3 m  open_orientation=fluids.thermal_liquid.valves.enum.orifice_orientation.positive  area_max=2.5e-5 m^2  area_leak=1e-10 m^2  S_TLU=[0, .002, .004, .007, .017] m  orifice_area_TLU=[1e-09, 2.0352e-07, 4.0736e-05, .00011438, .00034356] m^2  Cd=0.64  Re_c=150  smoothing_factor=0.01  pressure_recovery=false  S_flow_TLU=[0, .002, .004, .007, .017] m  p_diff_TLU=[.3, .5, .7] MPa  vol_flow_TLU=1e-3 * [1.7e-05, 2e-05, 2.6e-05; .0035, .0045, .0053; .7, .9, 1.06; 1.96, 2.5, 3; 6, 7.7, 9.13] m^3/s  mdot_TLU=[1.7e-05, 2e-05, 2.6e-05; .0035, .0045, .0053; .7, .9, 1.06; 1.96, 2.5, 3; 6, 7.7, 9.13] kg/s  T_ref_in=293.15 K  p_ref_in=0.101325 MPa  area=2.827e-5 m^2
      settings: InternalSimscapePortConfiguration="{\"Bottom\":[],\"Left\":[{\"id\":\"A\",\"label\":\"A\",\"type\":\"foundation.thermal_liquid.thermal_liquid\"},{\"id\":\"S\",\"label\":\"S\",\"type\":\"input\"}],\"Right\":[{\"id\":\"B\",\"label\":\"B\",\"type\":\"foundation.thermal_liquid.thermal_liquid\"}],\"Top\":[]}"
  hot_valve : SimscapeFluids_lib/Thermal Liquid/Valves & Orifices/Orifice (TL)  orifice_type=foundation.enum.constant_variable.variable  constant_orifice_spec=fluids.thermal_liquid.valves.enum.ConstantOrificeSpec.Area  variable_orifice_spec=fluids.thermal_liquid.valves.enum.orifice_spec.linear  orifice_area_constant=1e-3 m^2  p_diff_TLU_constant=[-4, -3, -2, -1, -.5, 0, .5, 1, 2, 3, 4] MPa  vol_flow_TLU_constant=[-2.44, -2.12, -1.68, -1.22, -.84, 0, .85, 1.21, 1.7, 2.09, 2.41] .* 1e-3 m^3/s  mdot_TLU_constant=[-2.44, -2.12, -1.68, -1.22, -.84, 0, .85, 1.21, 1.7, 2.09, 2.41] kg/s  S_min=0 m  del_S=5e-3 m  open_orientation=fluids.thermal_liquid.valves.enum.orifice_orientation.positive  area_max=2.5e-5 m^2  area_leak=1e-10 m^2  S_TLU=[0, .002, .004, .007, .017] m  orifice_area_TLU=[1e-09, 2.0352e-07, 4.0736e-05, .00011438, .00034356] m^2  Cd=0.64  Re_c=150  smoothing_factor=0.01  pressure_recovery=false  S_flow_TLU=[0, .002, .004, .007, .017] m  p_diff_TLU=[.3, .5, .7] MPa  vol_flow_TLU=1e-3 * [1.7e-05, 2e-05, 2.6e-05; .0035, .0045, .0053; .7, .9, 1.06; 1.96, 2.5, 3; 6, 7.7, 9.13] m^3/s  mdot_TLU=[1.7e-05, 2e-05, 2.6e-05; .0035, .0045, .0053; .7, .9, 1.06; 1.96, 2.5, 3; 6, 7.7, 9.13] kg/s  T_ref_in=293.15 K  p_ref_in=0.101325 MPa  area=2.827e-5 m^2
      settings: InternalSimscapePortConfiguration="{\"Bottom\":[],\"Left\":[{\"id\":\"A\",\"label\":\"A\",\"type\":\"foundation.thermal_liquid.thermal_liquid\"},{\"id\":\"S\",\"label\":\"S\",\"type\":\"input\"}],\"Right\":[{\"id\":\"B\",\"label\":\"B\",\"type\":\"foundation.thermal_liquid.thermal_liquid\"}],\"Top\":[]}"
  merged_flow : PMIOPort  Side=Right
  hot_valve_input : PMIOPort  Port=2  Side=Left
  hot_tap : PMIOPort  Port=3  Side=Left
  cold_supply : PMIOPort  Port=4  Side=Left
  cold_valve_input : PMIOPort  Port=5  Side=Left
  connections:
  hot_tap/RConn1 -- hot_valve/LConn1
  cold_supply/RConn1 -- cold_valve/LConn1
  hot_valve/LConn2 -- hot_valve_input/RConn1
  cold_valve/RConn1 -- merged_flow/RConn1 -- hot_valve/RConn1
  cold_valve/LConn2 -- cold_valve_input/RConn1

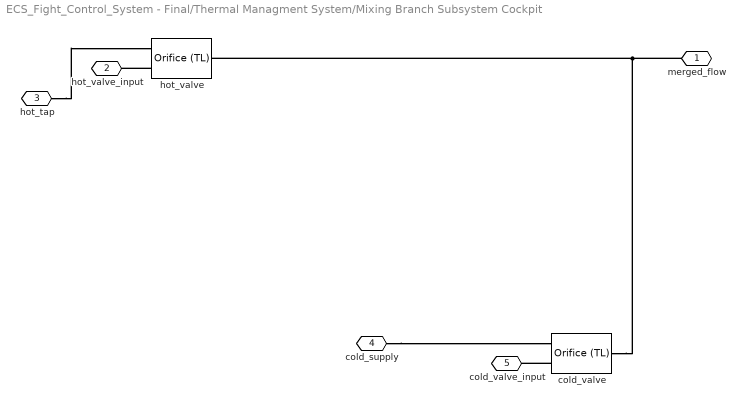
== system ECS_Fight_Control_System - Final/Thermal Managment System/Mixing Branch Subsystem Cockpit ==
  cold_valve : SimscapeFluids_lib/Thermal Liquid/Valves & Orifices/Orifice (TL)  orifice_type=foundation.enum.constant_variable.variable  constant_orifice_spec=fluids.thermal_liquid.valves.enum.ConstantOrificeSpec.Area  variable_orifice_spec=fluids.thermal_liquid.valves.enum.orifice_spec.linear  orifice_area_constant=1e-3 m^2  p_diff_TLU_constant=[-4, -3, -2, -1, -.5, 0, .5, 1, 2, 3, 4] MPa  vol_flow_TLU_constant=[-2.44, -2.12, -1.68, -1.22, -.84, 0, .85, 1.21, 1.7, 2.09, 2.41] .* 1e-3 m^3/s  mdot_TLU_constant=[-2.44, -2.12, -1.68, -1.22, -.84, 0, .85, 1.21, 1.7, 2.09, 2.41] kg/s  S_min=0 m  del_S=5e-3 m  open_orientation=fluids.thermal_liquid.valves.enum.orifice_orientation.positive  area_max=2.5e-5 m^2  area_leak=1e-10 m^2  S_TLU=[0, .002, .004, .007, .017] m  orifice_area_TLU=[1e-09, 2.0352e-07, 4.0736e-05, .00011438, .00034356] m^2  Cd=0.64  Re_c=150  smoothing_factor=0.01  pressure_recovery=false  S_flow_TLU=[0, .002, .004, .007, .017] m  p_diff_TLU=[.3, .5, .7] MPa  vol_flow_TLU=1e-3 * [1.7e-05, 2e-05, 2.6e-05; .0035, .0045, .0053; .7, .9, 1.06; 1.96, 2.5, 3; 6, 7.7, 9.13] m^3/s  mdot_TLU=[1.7e-05, 2e-05, 2.6e-05; .0035, .0045, .0053; .7, .9, 1.06; 1.96, 2.5, 3; 6, 7.7, 9.13] kg/s  T_ref_in=293.15 K  p_ref_in=0.101325 MPa  area=2.827e-5 m^2
      settings: InternalSimscapePortConfiguration="{\"Bottom\":[],\"Left\":[{\"id\":\"A\",\"label\":\"A\",\"type\":\"foundation.thermal_liquid.thermal_liquid\"},{\"id\":\"S\",\"label\":\"S\",\"type\":\"input\"}],\"Right\":[{\"id\":\"B\",\"label\":\"B\",\"type\":\"foundation.thermal_liquid.thermal_liquid\"}],\"Top\":[]}"
  hot_valve : SimscapeFluids_lib/Thermal Liquid/Valves & Orifices/Orifice (TL)  orifice_type=foundation.enum.constant_variable.variable  constant_orifice_spec=fluids.thermal_liquid.valves.enum.ConstantOrificeSpec.Area  variable_orifice_spec=fluids.thermal_liquid.valves.enum.orifice_spec.linear  orifice_area_constant=1e-3 m^2  p_diff_TLU_constant=[-4, -3, -2, -1, -.5, 0, .5, 1, 2, 3, 4] MPa  vol_flow_TLU_constant=[-2.44, -2.12, -1.68, -1.22, -.84, 0, .85, 1.21, 1.7, 2.09, 2.41] .* 1e-3 m^3/s  mdot_TLU_constant=[-2.44, -2.12, -1.68, -1.22, -.84, 0, .85, 1.21, 1.7, 2.09, 2.41] kg/s  S_min=0 m  del_S=5e-3 m  open_orientation=fluids.thermal_liquid.valves.enum.orifice_orientation.positive  area_max=2.5e-5 m^2  area_leak=1e-10 m^2  S_TLU=[0, .002, .004, .007, .017] m  orifice_area_TLU=[1e-09, 2.0352e-07, 4.0736e-05, .00011438, .00034356] m^2  Cd=0.64  Re_c=150  smoothing_factor=0.01  pressure_recovery=false  S_flow_TLU=[0, .002, .004, .007, .017] m  p_diff_TLU=[.3, .5, .7] MPa  vol_flow_TLU=1e-3 * [1.7e-05, 2e-05, 2.6e-05; .0035, .0045, .0053; .7, .9, 1.06; 1.96, 2.5, 3; 6, 7.7, 9.13] m^3/s  mdot_TLU=[1.7e-05, 2e-05, 2.6e-05; .0035, .0045, .0053; .7, .9, 1.06; 1.96, 2.5, 3; 6, 7.7, 9.13] kg/s  T_ref_in=293.15 K  p_ref_in=0.101325 MPa  area=2.827e-5 m^2
      settings: InternalSimscapePortConfiguration="{\"Bottom\":[],\"Left\":[{\"id\":\"A\",\"label\":\"A\",\"type\":\"foundation.thermal_liquid.thermal_liquid\"},{\"id\":\"S\",\"label\":\"S\",\"type\":\"input\"}],\"Right\":[{\"id\":\"B\",\"label\":\"B\",\"type\":\"foundation.thermal_liquid.thermal_liquid\"}],\"Top\":[]}"
  merged_flow : PMIOPort  Side=Right
  hot_valve_input : PMIOPort  Port=2  Side=Left
  hot_tap : PMIOPort  Port=3  Side=Left
  cold_supply : PMIOPort  Port=4  Side=Left
  cold_valve_input : PMIOPort  Port=5  Side=Left
  connections:
  hot_tap/RConn1 -- hot_valve/LConn1
  cold_supply/RConn1 -- cold_valve/LConn1
  hot_valve/LConn2 -- hot_valve_input/RConn1
  cold_valve/RConn1 -- hot_valve/RConn1 -- merged_flow/RConn1
  cold_valve/LConn2 -- cold_valve_input/RConn1

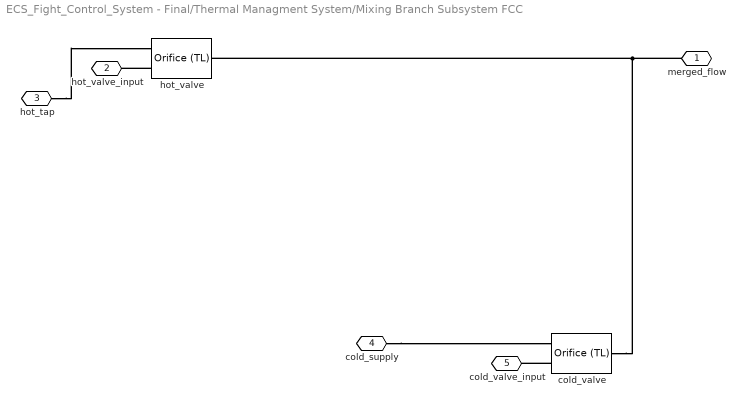
== system ECS_Fight_Control_System - Final/Thermal Managment System/Mixing Branch Subsystem FCC ==
  cold_valve : SimscapeFluids_lib/Thermal Liquid/Valves & Orifices/Orifice (TL)  orifice_type=foundation.enum.constant_variable.variable  constant_orifice_spec=fluids.thermal_liquid.valves.enum.ConstantOrificeSpec.Area  variable_orifice_spec=fluids.thermal_liquid.valves.enum.orifice_spec.linear  orifice_area_constant=1e-3 m^2  p_diff_TLU_constant=[-4, -3, -2, -1, -.5, 0, .5, 1, 2, 3, 4] MPa  vol_flow_TLU_constant=[-2.44, -2.12, -1.68, -1.22, -.84, 0, .85, 1.21, 1.7, 2.09, 2.41] .* 1e-3 m^3/s  mdot_TLU_constant=[-2.44, -2.12, -1.68, -1.22, -.84, 0, .85, 1.21, 1.7, 2.09, 2.41] kg/s  S_min=0 m  del_S=5e-3 m  open_orientation=fluids.thermal_liquid.valves.enum.orifice_orientation.positive  area_max=2.5e-5 m^2  area_leak=1e-10 m^2  S_TLU=[0, .002, .004, .007, .017] m  orifice_area_TLU=[1e-09, 2.0352e-07, 4.0736e-05, .00011438, .00034356] m^2  Cd=0.64  Re_c=150  smoothing_factor=0.01  pressure_recovery=false  S_flow_TLU=[0, .002, .004, .007, .017] m  p_diff_TLU=[.3, .5, .7] MPa  vol_flow_TLU=1e-3 * [1.7e-05, 2e-05, 2.6e-05; .0035, .0045, .0053; .7, .9, 1.06; 1.96, 2.5, 3; 6, 7.7, 9.13] m^3/s  mdot_TLU=[1.7e-05, 2e-05, 2.6e-05; .0035, .0045, .0053; .7, .9, 1.06; 1.96, 2.5, 3; 6, 7.7, 9.13] kg/s  T_ref_in=293.15 K  p_ref_in=0.101325 MPa  area=2.827e-5 m^2
      settings: InternalSimscapePortConfiguration="{\"Bottom\":[],\"Left\":[{\"id\":\"A\",\"label\":\"A\",\"type\":\"foundation.thermal_liquid.thermal_liquid\"},{\"id\":\"S\",\"label\":\"S\",\"type\":\"input\"}],\"Right\":[{\"id\":\"B\",\"label\":\"B\",\"type\":\"foundation.thermal_liquid.thermal_liquid\"}],\"Top\":[]}"
  hot_valve : SimscapeFluids_lib/Thermal Liquid/Valves & Orifices/Orifice (TL)  orifice_type=foundation.enum.constant_variable.variable  constant_orifice_spec=fluids.thermal_liquid.valves.enum.ConstantOrificeSpec.Area  variable_orifice_spec=fluids.thermal_liquid.valves.enum.orifice_spec.linear  orifice_area_constant=1e-3 m^2  p_diff_TLU_constant=[-4, -3, -2, -1, -.5, 0, .5, 1, 2, 3, 4] MPa  vol_flow_TLU_constant=[-2.44, -2.12, -1.68, -1.22, -.84, 0, .85, 1.21, 1.7, 2.09, 2.41] .* 1e-3 m^3/s  mdot_TLU_constant=[-2.44, -2.12, -1.68, -1.22, -.84, 0, .85, 1.21, 1.7, 2.09, 2.41] kg/s  S_min=0 m  del_S=5e-3 m  open_orientation=fluids.thermal_liquid.valves.enum.orifice_orientation.positive  area_max=2.5e-5 m^2  area_leak=1e-10 m^2  S_TLU=[0, .002, .004, .007, .017] m  orifice_area_TLU=[1e-09, 2.0352e-07, 4.0736e-05, .00011438, .00034356] m^2  Cd=0.64  Re_c=150  smoothing_factor=0.01  pressure_recovery=false  S_flow_TLU=[0, .002, .004, .007, .017] m  p_diff_TLU=[.3, .5, .7] MPa  vol_flow_TLU=1e-3 * [1.7e-05, 2e-05, 2.6e-05; .0035, .0045, .0053; .7, .9, 1.06; 1.96, 2.5, 3; 6, 7.7, 9.13] m^3/s  mdot_TLU=[1.7e-05, 2e-05, 2.6e-05; .0035, .0045, .0053; .7, .9, 1.06; 1.96, 2.5, 3; 6, 7.7, 9.13] kg/s  T_ref_in=293.15 K  p_ref_in=0.101325 MPa  area=2.827e-5 m^2
      settings: InternalSimscapePortConfiguration="{\"Bottom\":[],\"Left\":[{\"id\":\"A\",\"label\":\"A\",\"type\":\"foundation.thermal_liquid.thermal_liquid\"},{\"id\":\"S\",\"label\":\"S\",\"type\":\"input\"}],\"Right\":[{\"id\":\"B\",\"label\":\"B\",\"type\":\"foundation.thermal_liquid.thermal_liquid\"}],\"Top\":[]}"
  merged_flow : PMIOPort  Side=Right
  hot_valve_input : PMIOPort  Port=2  Side=Left
  hot_tap : PMIOPort  Port=3  Side=Left
  cold_supply : PMIOPort  Port=4  Side=Left
  cold_valve_input : PMIOPort  Port=5  Side=Left
  connections:
  cold_valve/LConn2 -- cold_valve_input/RConn1
  merged_flow/RConn1 -- hot_valve/RConn1 -- cold_valve/RConn1
  hot_valve/LConn2 -- hot_valve_input/RConn1
  cold_supply/RConn1 -- cold_valve/LConn1
  hot_tap/RConn1 -- hot_valve/LConn1

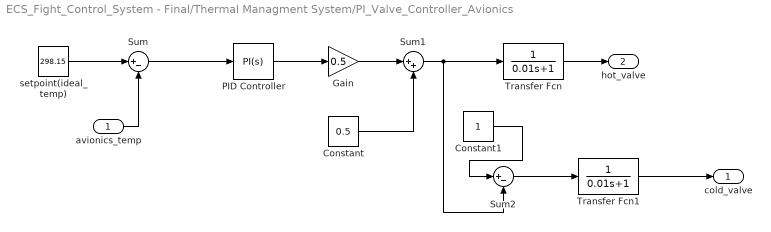
== system ECS_Fight_Control_System - Final/Thermal Managment System/PI_Valve_Controller_Avionics ==
  avionics_temp : Inport
  Constant : Constant  Value=0.5
  Constant1 : Constant
  Gain : Gain  Gain=0.5
  PID Controller : slpidlib/PID Controller  Controller=PI  Form=Parallel  TimeDomain=Continuous-time  UseExternalTs=off  SampleTime=-1  IntegratorMethod=Forward Euler  FilterMethod=Forward Euler  ControllerParametersSource=internal  P=0.5  I=0.1  UseKiTs=off  D=0  UseExternalDerivativeSource=off  N=100  UseFilter=on  TunerSelectOption=Transfer Function Based (PID Tuner App)  InitialConditionSource=internal  InitialConditionForIntegrator=0  InitialConditionForFilter=0  DifferentiatorICPrevScaledInput=0  ExternalReset=none  TrackingMode=off  Kt=1  LimitOutput=on  SatLimitsSource=internal  UpperSaturationLimit=1  LowerSaturationLimit=-1  LinearizeAsGain=on  AntiWindupMode=clamping  Kb=1  LimitIntegrator=off  UpperIntegratorSaturationLimit=inf  LowerIntegratorSaturationLimit=-inf  POutMin=[]  POutMax=[]  IOutMin=[]  IOutMax=[]  DOutMin=[]  DOutMax=[]  NOutMin=[]  NOutMax=[]  SumOutMin=[]  SumOutMax=[]  SaturationOutMin=[]  SaturationOutMax=[]  PParamMin=[]  PParamMax=[]  IParamMin=[]  IParamMax=[]  DParamMin=[]  DParamMax=[]  NParamMin=[]  NParamMax=[]  KbParamMin=[]  KbParamMax=[]  KtParamMin=[]  KtParamMax=[]  KbOutMin=[]  KbOutMax=[]  KtOutMin=[]  KtOutMax=[]  IntegratorOutMin=[]  IntegratorOutMax=[]  FilterOutMin=[]  FilterOutMax=[]  SumI1OutMin=[]  SumI1OutMax=[]  SumI2OutMin=[]  SumI2OutMax=[]  SumI3OutMin=[]  SumI3OutMax=[]  SumI4OutMin=[]  SumI4OutMax=[]  SumDOutMin=[]  SumDOutMax=[]  DifferentiatorOutMin=[]  DifferentiatorOutMax=[]  FilterDiffOutCoefMin=[]  FilterDiffOutCoefMax=[]  ReciprocalOutMin=[]  ReciprocalOutMax=[]  SumDenOutMin=[]  SumDenOutMax=[]  SumNumOutMin=[]  SumNumOutMax=[]  DivideOutMin=[]  DivideOutMax=[]  UdiffTsProdOutMin=[]  UdiffTsProdOutMax=[]  NTsProdOutMin=[]  NTsProdOutMax=[]  UintegralTsProdOutMin=[]  UintegralTsProdOutMax=[]  UngainTsProdOutMin=[]  UngainTsProdOutMax=[]  ClampingZeroOutDataTypeStr=Inherit: Inherit via back propagation  ClampingZeroOutMin=[]  ClampingZeroOutMax=[]  FilterDenConstantOutDataTypeStr=Inherit: Inherit via back propagation  FilterDenConstantOutMin=[]  FilterDenConstantOutMax=[]  PCopyOutDataTypeStr=Inherit: Inherit via back propagation  PCopyOutMin=[]  PCopyOutMax=[]  NCopyOutDataTypeStr=Inherit: Inherit via back propagation  NCopyOutMin=[]  NCopyOutMax=[]  IntegratorContinuousStateAttributes=''  IntegratorStateMustResolveToSignalObject=off  IntegratorRTWStateStorageClass=Auto  FilterContinuousStateAttributes=''  FilterStateMustResolveToSignalObject=off  FilterRTWStateStorageClass=Auto  ParallelPVariant=InternalParameters  IdealPVariant=Disabled  IVariant=InternalParameters  DVariant=Disabled  IntegratorVariant=Continuous  SatVariant=Enabled  AWVariant=ContClampingParallel  PCopyVariant=Disabled  TRVariant=Disabled  FdbkBlocksVariant=Forward  IdealPFdbkVariant=Disabled  SatFdbkVariant=Disabled  DerivativeFilterVariant=Disabled  NVariant=Disabled  NCopyVariant=Disabled_SignalSpec  FilterICVariant=Disabled  IntegratorICVariant=InternalICs  ExternalResetVariant=Disabled  TRSumVariant=Passthrough  SumFdbkVariant=Disabled  SumVariant=Sum_PI  TsampFilterVariant=InternalTs  TsampNgainVariant=Passthrough  TsampIntegralVariant=Disabled_SignalSpec  ExternalSaturationOutDataTypeStr=Inherit: Same as second input  DerivativeSourceVariant=Disabled  PreIntVariant=InternalPreInt
  Sum : Sum  Inputs=|+-
  Sum1 : Sum  Inputs=|++
  Sum2 : Sum  Inputs=|+-
  Transfer Fcn : TransferFcn  Denominator=[0.01 1]
  Transfer Fcn1 : TransferFcn  Denominator=[0.01 1]
  setpoint(ideal_temp) : Constant  Value=298.15
  cold_valve : Outport
  hot_valve : Outport  Port=2
  wires:
  PID Controller/1 -> Gain/1
  Sum/1 -> PID Controller/1
  setpoint(ideal_temp)/1 -> Sum/1
  avionics_temp/1 -> Sum/2
  Gain/1 -> Sum1/1
  Constant/1 -> Sum1/2
  Sum1/1 -> Sum2/2, Transfer Fcn/1
  Constant1/1 -> Sum2/1
  Sum2/1 -> Transfer Fcn1/1
  Transfer Fcn/1 -> hot_valve/1
  Transfer Fcn1/1 -> cold_valve/1
